simulink model "Evita_paredes"  (R2023b)
settings: Solver=VariableStepAuto  StartTime=0.0  StopTime=10.0  RelTol=1e-3
libraries: arduinolib x11, simulink x7
settings Model: Creator=alber  LastModifiedBy=alber

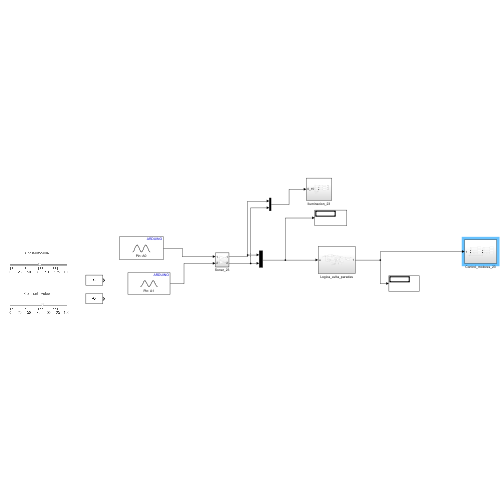
[thumbnail: Simulink's stored preview of the top-level diagram]
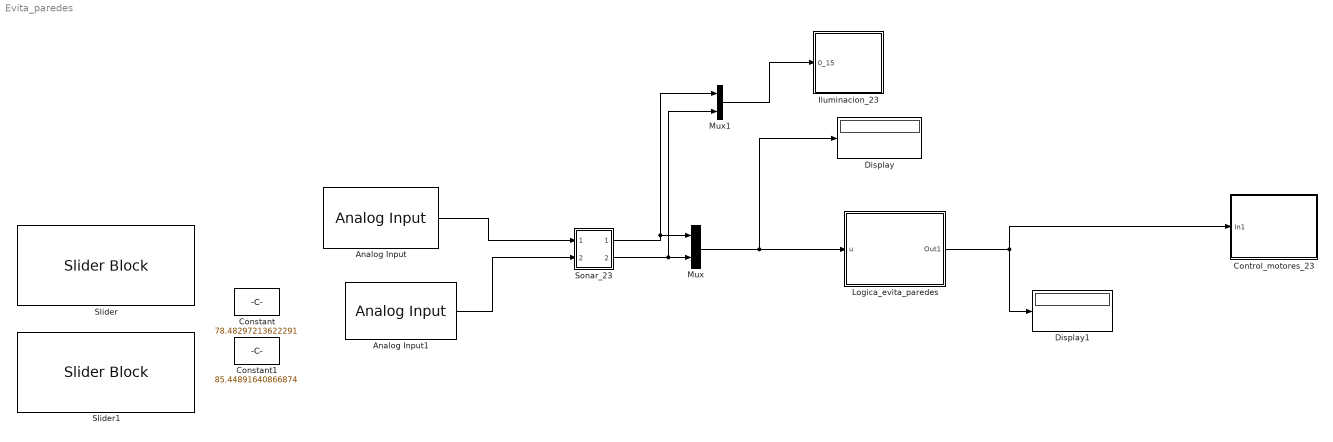
== system Evita_paredes ==
  Analog Input : arduinolib/Analog Input  pinNumber=0  ReadResultsOnly=off  ConversionTriggerSource=Software  ExternalTriggerType=uint32( 0 )  OutputDataType=uint16  EnableConversionCompleteNotify=off  EnableOuputStatus=off  SampleTime=-1  blockPlatform=arduino
  Analog Input1 : arduinolib/Analog Input  pinNumber=1  ReadResultsOnly=off  ConversionTriggerSource=Software  ExternalTriggerType=uint32( 0 )  OutputDataType=uint16  EnableConversionCompleteNotify=off  EnableOuputStatus=off  SampleTime=-1  blockPlatform=arduino
  Constant : Constant  Value=78.48297213622291
  Constant1 : Constant  Value=85.44891640866874
  Control_motores_23 : Subsystem
  Display : Display
  Display1 : Display
  Iluminacion_23 : Subsystem
  Logica_evita_paredes : Subsystem
  Mux : Mux  Inputs=2
  Mux1 : Mux  Inputs=2
  Slider : SliderBlock  ScaleMax=150
  Slider1 : SliderBlock  ScaleMax=150
  Sonar_23 : Subsystem
  wires:
  Analog Input/1 -> Sonar_23/1(In1)
  Logica_evita_paredes/1(Out1) -> Control_motores_23/1(In1), Display1/1
  Analog Input1/1 -> Sonar_23/2(In2)
  Sonar_23/2(Out2) -> Mux1/2, Mux/2
  Mux1/1 -> Iluminacion_23/1(0_15)
  Mux/1 -> Logica_evita_paredes/1(u), Display/1
  Sonar_23/1(Out1) -> Mux1/1, Mux/1

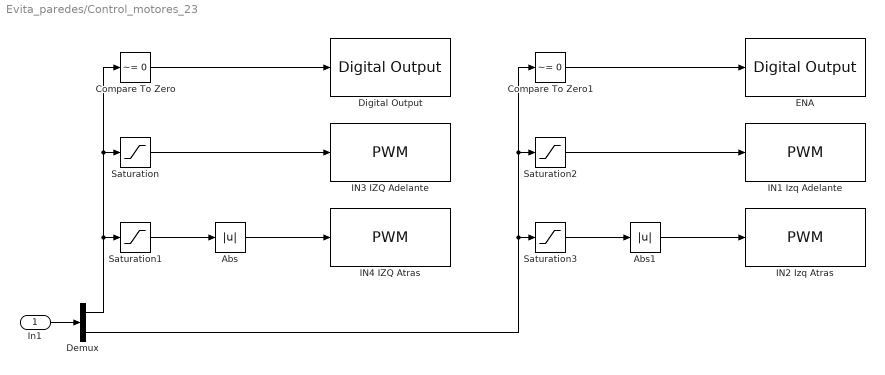
== system Evita_paredes/Control_motores_23 ==
  In1 : Inport  OutMin=[0]  OutMax=[255]  PortDimensions=2
  Abs : Abs  SaturateOnIntegerOverflow=off
  Abs1 : Abs  SaturateOnIntegerOverflow=off
  Compare To Zero : simulink/Logic and Bit Operations/Compare To Zero  relop=~=  OutDataTypeStr=boolean
  Compare To Zero1 : simulink/Logic and Bit Operations/Compare To Zero  relop=~=  OutDataTypeStr=boolean
  Demux : Demux  Outputs=2
  Digital Output : arduinolib/Digital Output  pinNumber=13  Direction=output  blockPlatform=arduino
  ENA : arduinolib/Digital Output  pinNumber=8  Direction=output  blockPlatform=arduino
  IN1 Izq Adelante : arduinolib/PWM  pinNumber=9  frequencyType=Default  desiredFrequency=490.2  achievableFrequency=490.2
  IN2 Izq Atras : arduinolib/PWM  pinNumber=10  frequencyType=Default  desiredFrequency=490.2  achievableFrequency=490.2
  IN3 IZQ Adelante : arduinolib/PWM  pinNumber=11  frequencyType=Default  desiredFrequency=490.2  achievableFrequency=490.2
  IN4 IZQ Atras : arduinolib/PWM  pinNumber=12  frequencyType=Default  desiredFrequency=490.2  achievableFrequency=490.2
  Saturation : Saturate  UpperLimit=255  LowerLimit=0
  Saturation1 : Saturate  UpperLimit=0  LowerLimit=-255
  Saturation2 : Saturate  UpperLimit=255  LowerLimit=0
  Saturation3 : Saturate  UpperLimit=0  LowerLimit=-255
  wires:
  Demux/2 -> Compare To Zero1/1, Saturation2/1, Saturation3/1
  Demux/1 -> Compare To Zero/1, Saturation/1, Saturation1/1
  Saturation3/1 -> Abs1/1
  Saturation2/1 -> IN1 Izq Adelante/1
  Compare To Zero/1 -> Digital Output/1
  Abs/1 -> IN4 IZQ Atras/1
  Abs1/1 -> IN2 Izq Atras/1
  Compare To Zero1/1 -> ENA/1
  In1/1 -> Demux/1
  Saturation1/1 -> Abs/1
  Saturation/1 -> IN3 IZQ Adelante/1

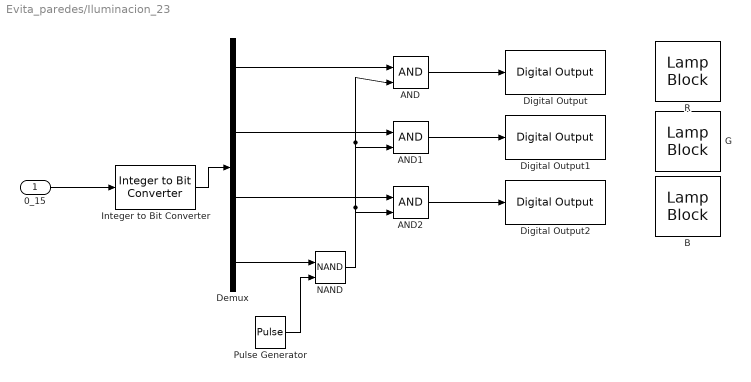
== system Evita_paredes/Iluminacion_23 ==
  0_15 : Inport
  AND : Logic  IconShape=distinctive  AllPortsSameDT=off  OutDataTypeStr=boolean
  AND1 : Logic  IconShape=distinctive  AllPortsSameDT=off  OutDataTypeStr=boolean
  AND2 : Logic  IconShape=distinctive  AllPortsSameDT=off  OutDataTypeStr=boolean
  B : LampBlock  LabelPosition=Hide
  Demux : Demux
  Digital Output : arduinolib/Digital Output  pinNumber=49  Direction=output  blockPlatform=arduino
  Digital Output1 : arduinolib/Digital Output  pinNumber=51  Direction=output  blockPlatform=arduino
  Digital Output2 : arduinolib/Digital Output  pinNumber=53  Direction=output  blockPlatform=arduino
  G : LampBlock  LabelPosition=Hide
  Integer to Bit Converter : simulink/Logic and Bit Operations/Integer to Bit Converter  nbits=4  signedInputValues=Unsigned  bitOrder=LSB first  outDtype=boolean
  NAND : Logic  Operator=NAND  IconShape=distinctive  AllPortsSameDT=off  OutDataTypeStr=boolean
  Pulse Generator : DiscretePulseGenerator  PulseType=Time based  Period=1  PulseWidth=50
  R : LampBlock  LabelPosition=Hide
  wires:
  Demux/1 -> AND/1
  NAND/1 -> AND2/2, AND1/2, AND/2
  AND2/1 -> Digital Output2/1
  Demux/2 -> AND1/1
  Integer to Bit Converter/1 -> Demux/1
  AND1/1 -> Digital Output1/1
  Demux/3 -> AND2/1
  AND/1 -> Digital Output/1
  Demux/4 -> NAND/1
  0_15/1 -> Integer to Bit Converter/1
  Pulse Generator/1 -> NAND/2

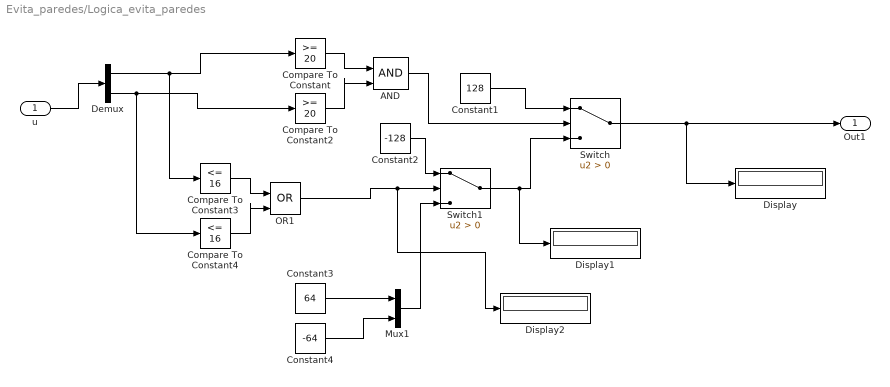
== system Evita_paredes/Logica_evita_paredes ==
  u : Inport
  AND : Logic  IconShape=distinctive  AllPortsSameDT=off  OutDataTypeStr=boolean
  Compare To Constant : simulink/Logic and Bit Operations/Compare To Constant  relop=>=  const=20  OutDataTypeStr=uint8
  Compare To Constant2 : simulink/Logic and Bit Operations/Compare To Constant  relop=>=  const=20  OutDataTypeStr=uint8
  Compare To Constant3 : simulink/Logic and Bit Operations/Compare To Constant  relop=<=  const=16  OutDataTypeStr=uint8
  Compare To Constant4 : simulink/Logic and Bit Operations/Compare To Constant  relop=<=  const=16  OutDataTypeStr=uint8
  Constant1 : Constant  Value=128
  Constant2 : Constant  Value=-128
  Constant3 : Constant  Value=64
  Constant4 : Constant  Value=-64
  Demux : Demux  Outputs=2
  Display : Display
  Display1 : Display
  Display2 : Display
  Mux1 : Mux  Inputs=2
  OR1 : Logic  Operator=OR  IconShape=distinctive  AllPortsSameDT=off
  Switch : Switch  Criteria=u2 > Threshold  SaturateOnIntegerOverflow=off  InputSameDT=off
  Switch1 : Switch  Criteria=u2 > Threshold  SaturateOnIntegerOverflow=off  InputSameDT=off
  Out1 : Outport
  wires:
  Compare To Constant3/1 -> OR1/1
  Constant2/1 -> Switch1/1
  Constant4/1 -> Mux1/2
  Switch1/1 -> Display1/1, Switch/3
  Demux/2 -> Compare To Constant4/1, Compare To Constant2/1
  Demux/1 -> Compare To Constant/1, Compare To Constant3/1
  Constant1/1 -> Switch/1
  OR1/1 -> Switch1/2, Display2/1
  u/1 -> Demux/1
  Compare To Constant/1 -> AND/1
  AND/1 -> Switch/2
  Switch/1 -> Out1/1, Display/1
  Compare To Constant2/1 -> AND/2
  Constant3/1 -> Mux1/1
  Compare To Constant4/1 -> OR1/2
  Mux1/1 -> Switch1/3

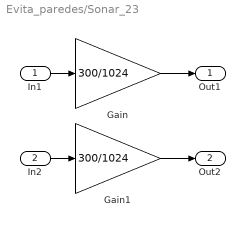
== system Evita_paredes/Sonar_23 ==
  In1 : Inport
  In2 : Inport  Port=2
  Gain : Gain  Gain=300/1024
  Gain1 : Gain  Gain=300/1024
  Out1 : Outport
  Out2 : Outport  Port=2
  wires:
  Gain/1 -> Out1/1
  In1/1 -> Gain/1
  In2/1 -> Gain1/1
  Gain1/1 -> Out2/1
